simulink model "TGWH3"  (R2019b)
settings: Solver=ode45  StartTime=0.0  StopTime=10  MaxStep=1  RelTol=1e-3
values from neighbouring files (symbols this model uses):
  Cpm = 385    [main.m]
  Cpw = 4186    [main.m]
  DeltaTin = 0.75    [main.m]
  DeltaTout = 0.75    [main.m]
  flow_rate_input = flow_signal(k)    [main.m]
  Li = 2.2    [main.m]
  Mm = 2    [main.m]
  Mw = 2    [main.m]
  Power_delay = 2.5    [main.m]
  Power_input = u(1)    [main.m]
  Power_max = 58300    [main.m]
  ri = 8e-3    (= 0.008)    [main.m]
  ro = 1000    [main.m]
  T_in = 15    [main.m]
settings Model: Creator=and88  LastModifiedBy=and88
settings DataIOCC: FinalStateName=myOperPoint  InitialState=myOperPoint

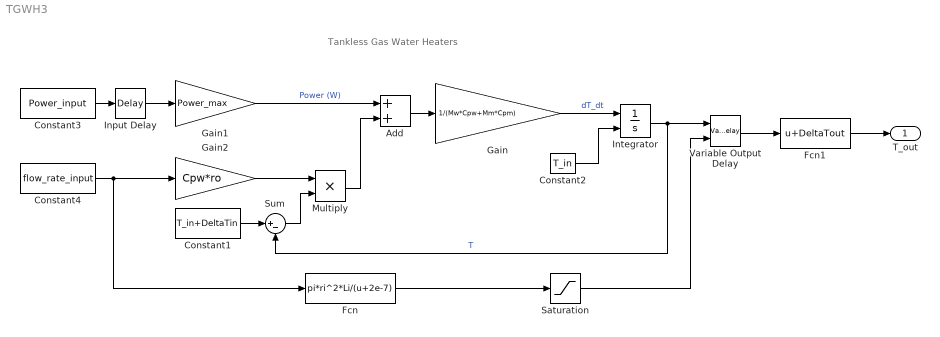
== system TGWH3 ==
  note: Tankless Gas Water Heaters
  Add : Sum
  Constant1 : Constant  Value=T_in+DeltaTin
  Constant2 : Constant  Value=T_in
  Constant3 : Constant  Value=Power_input
  Constant4 : Constant  Value=flow_rate_input
  Fcn : Fcn  Expr=pi*ri^2*Li/(u+2e-7)
  Fcn1 : Fcn  Expr=u+DeltaTout
  Gain : Gain  Gain=1/(Mw*Cpw+Mm*Cpm)
  Gain1 : Gain  Gain=Power_max
  Gain2 : Gain  Gain=Cpw*ro
  Input Delay : TransportDelay  DelayTime=Power_delay  BufferSize=11264
  Integrator : Integrator  InitialConditionSource=external
  Multiply : Product
  Saturation : Saturate  UpperLimit=10  LowerLimit=0  LinearizeAsGain=off
  Sum : Sum  Inputs=|+-
  Variable Output Delay : VariableTransportDelay  MaximumDelay=10  InitialOutput=T_in  MaximumPoints=11264
  T_out : Outport  VectorParamsAs1DForOutWhenUnconnected=off
  wires:
  Constant1/1 -> Sum/1
  Sum/1 -> Multiply/2
  Multiply/1 -> Add/2
  Constant2/1 -> Integrator/2
  Fcn1/1 -> T_out/1
  Gain2/1 -> Multiply/1
  Add/1 -> Gain/1
  Gain1/1 -> Add/1  "Power (W)"
  Gain/1 -> Integrator/1  "dT_dt"
  Constant4/1 -> Gain2/1, Fcn/1
  Integrator/1 -> Variable Output Delay/1, Sum/2  "T"
  Constant3/1 -> Input Delay/1
  Input Delay/1 -> Gain1/1
  Fcn/1 -> Saturation/1
  Saturation/1 -> Variable Output Delay/2
  Variable Output Delay/1 -> Fcn1/1
